simulink model "Task_4_Without_Feedback"  (R2018a)
settings: Solver=VariableStepAuto  StartTime=0.0  StopTime=10.0  MaxStep=0.001  RelTol=1e-3
libraries: simulink x2
settings Model: Creator=HP  LastModifiedBy=HP

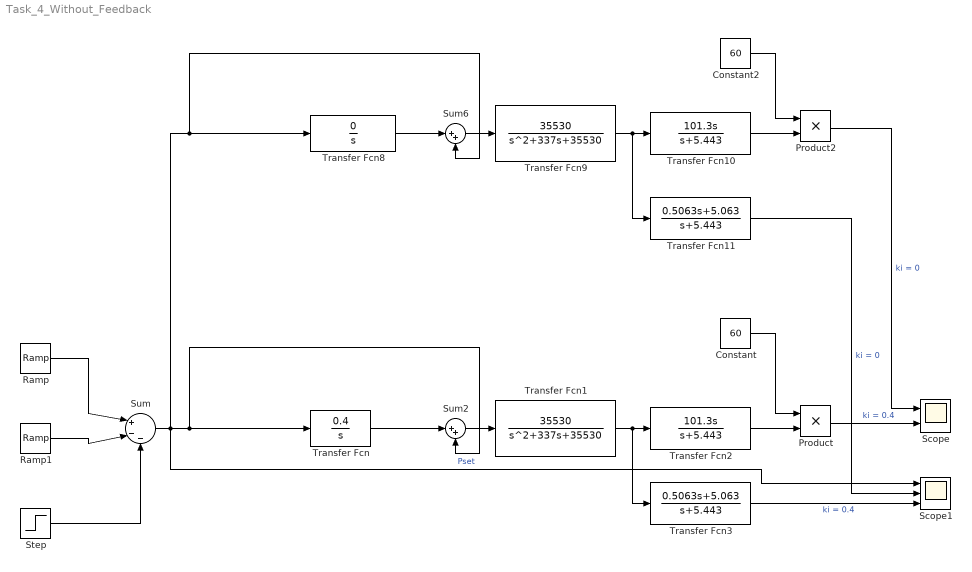
== system Task_4_Without_Feedback ==
  Constant : Constant  Value=60
  Constant2 : Constant  Value=60
  Product : Product
  Product2 : Product
  Ramp : simulink/Sources/Ramp  slope=64.9351  start=1  InitialOutput=0
  Ramp1 : simulink/Sources/Ramp  slope=64.9531  start=1.231  InitialOutput=0
  Scope : Scope  NumInputPorts=2
  Scope1 : Scope  NumInputPorts=3
  Step : Step  Time=5  After=15  SampleTime=0
  Sum : Sum  Inputs=|+--
  Sum2 : Sum  Inputs=|++
  Sum6 : Sum  Inputs=|++
  Transfer Fcn : TransferFcn  Numerator=[0.4]  Denominator=[1 0]
  Transfer Fcn1 : TransferFcn  Numerator=[35530]  Denominator=[1 337 35530]
  Transfer Fcn10 : TransferFcn  Numerator=[101.3 0]  Denominator=[1 5.443]
  Transfer Fcn11 : TransferFcn  Numerator=[0.5063 5.063]  Denominator=[1 5.443]
  Transfer Fcn2 : TransferFcn  Numerator=[101.3 0]  Denominator=[1 5.443]
  Transfer Fcn3 : TransferFcn  Numerator=[0.5063 5.063]  Denominator=[1 5.443]
  Transfer Fcn8 : TransferFcn  Numerator=[0]  Denominator=[1 0]
  Transfer Fcn9 : TransferFcn  Numerator=[35530]  Denominator=[1 337 35530]
  wires:
  Ramp1/1 -> Sum/2
  Step/1 -> Sum/3
  Transfer Fcn1/1 -> Transfer Fcn3/1, Transfer Fcn2/1
  Sum2/1 -> Transfer Fcn1/1
  Constant/1 -> Product/1
  Transfer Fcn3/1 -> Scope1/3  "ki = 0.4"
  Sum/1 -> Scope1/1, Sum6/2, Transfer Fcn8/1, Transfer Fcn/1, Sum2/2  "Pset"
  Transfer Fcn2/1 -> Product/2
  Transfer Fcn/1 -> Sum2/1
  Transfer Fcn8/1 -> Sum6/1
  Transfer Fcn11/1 -> Scope1/2  "ki = 0"
  Product/1 -> Scope/2  "ki = 0.4"
  Constant2/1 -> Product2/1
  Ramp/1 -> Sum/1
  Transfer Fcn9/1 -> Transfer Fcn11/1, Transfer Fcn10/1
  Sum6/1 -> Transfer Fcn9/1
  Transfer Fcn10/1 -> Product2/2
  Product2/1 -> Scope/1  "ki = 0"
